simulink model "PQ_Control_LCL_4Legs"  (R2023b)
settings: Solver=FixedStepAuto  StartTime=0.0  StopTime=10.0  RelTol=1e-3
InitFcn:
  | Initialization_for_PQ_Control_LCL_4Legs;
values from neighbouring files (symbols this model uses):
  Fnom_Grid = 50    [Initialization_for_PQ_Control_LCL_4Legs.m]
  Gain_for_ActiveDamping = 1    [Initialization_for_PQ_Control_LCL_4Legs.m]
  Inom = Pnom/sqrt(3)/Unom_Grid    [Initialization_for_PQ_Control_LCL_4Legs.m]
  Ki_Idq = Kp_Idq*2*pi*0.5    (= 6.3165468167)    [Initialization_for_PQ_Control_LCL_4Legs.m]
  Ki_Un = Cdc/L_neutral*Kp_Un^2*Udc_ref/Inom    [Initialization_for_PQ_Control_LCL_4Legs.m]
  Kp_Idq = L_grid*2*pi*1600    (= 2.0106192983)    [Initialization_for_PQ_Control_LCL_4Legs.m]
  Kp_Un = 2*pi*Fnom_Grid*L_neutral*10    (= 1.13097335529)    [Initialization_for_PQ_Control_LCL_4Legs.m]
  L_grid = 200e-6    (= 0.0002)    [Initialization_for_PQ_Control_LCL_4Legs.m]
  Ts_Control = 62.5e-6    (= 6.25e-05)    [Initialization_for_PQ_Control_LCL_4Legs.m]
  Udc_ref = 1500    [Initialization_for_PQ_Control_LCL_4Legs.m]
  Unom_Phase = Unom_Grid/sqrt(3)    [Initialization_for_PQ_Control_LCL_4Legs.m]
libraries: LibraryForCodeGeneration x14
settings Model: DataDictionary=VariablesDictionary_for_PQ_Control_LCL_4Legs.sldd  TunableVars=Inom,Ki_Idq,Kp_Idq,Udc_ref,Unom_Phase  TunableVarsStorageClass=Auto,Auto,Auto,Auto,Auto  TunableVarsTypeQualifier=,,,,  Creator=ZZY  LastModifiedBy=ZZY
settings OptimizationCC: BlockReduction=off  DefaultParameterBehavior=Inlined  UseDivisionForNetSlopeComputation=on  ReuseModelBlockBuffer=off  ExpressionFolding=off  PassReuseOutputArgsAs=Individual arguments  ZeroExternalMemoryAtStartup=off  ZeroInternalMemoryAtStartup=off  EfficientFloat2IntCast=on  LifeSpan=inf  OptimizationLevel=level1  LabelGuidedReuse=on  EfficientTunableParamExpr=on
settings DebuggingCC: SignalInfNanChecking=warning  SignalRangeChecking=warning  ReadBeforeWriteMsg=EnableAllAsError  WriteAfterWriteMsg=EnableAllAsError  WriteAfterReadMsg=EnableAllAsError  IntegerOverflowMsg=error  ParameterPrecisionLossMsg=none  FixptConstUnderflowMsg=warning  FixptConstOverflowMsg=warning  FixptConstPrecisionLossMsg=warning  UnnecessaryDatatypeConvMsg=warning  UniqueDataStoreMsg=error  AssertControl=DisableAll  NonBusSignalsTreatedAsBus=error  SFInvalidInputDataAccessInChartInitDiag=error  SFTransitionOutsideNaturalParentDiag=error  SFUnreachableExecutionPathDiag=error  SFUndirectedBroadcastEventsDiag=error  IntegerSaturationMsg=error
settings HardwareCC: ProdBitPerChar=16  ProdBitPerInt=16  ProdBitPerPointer=32  ProdBitPerSizeT=32  ProdBitPerPtrDiffT=32  ProdLargestAtomicInteger=Integer  ProdLargestAtomicFloat=None  ProdWordSize=16  ProdHWDeviceType=Texas Instruments->C2000  TargetBitPerChar=16  TargetBitPerInt=16  TargetLargestAtomicInteger=Integer  TargetIntDivRoundTo=Zero  TargetEndianess=LittleEndian  TargetWordSize=16  TargetHWDeviceType=Texas Instruments->C2000
settings SFSimCC: CompileTimeRecursionLimit=0  EnableRuntimeRecursion=off  MATLABDynamicMemAlloc=off
settings RTWCC: Description=Embedded Coder  SystemTargetFile=ert.tlc  TemplateMakefile=ert_default_tmf  GenerateReport=on  Toolchain=MinGW64 | gmake (64-bit Windows)  BuildConfiguration=Faster Runs  IncludeHyperlinkInReport=on  LaunchReport=on  DataTypeReplacement=CDataTypesFixedWidth  GenerateTraceInfo=on  GenerateTraceReport=on  GenerateTraceReportSl=on  GenerateTraceReportSf=on  GenerateTraceReportEml=on  GenerateWebview=on  GenerateCodeReplacementReport=on  CheckMdlBeforeBuild=Warning
settings CodeAppCC: ForceParamTrailComments=on  IgnoreCustomStorageClasses=off  OperatorAnnotations=on  SimulinkDataObjDesc=on  SFDataObjDesc=on  MATLABFcnDesc=on  DefineNamingRule=UpperCase  InsertBlockDesc=on  StateflowObjectComments=on  MATLABSourceComments=on  InlinedPrmAccess=Macros  ReqsInCode=on
settings ERTTargetCC: TargetLangStandard=C99 (ISO)  GenerateSampleERTMain=on  CombineSignalStateStructs=on  GroupInternalDataByFunction=on  ParenthesesLevel=Standards  CastingMode=Standards  GenerateSharedConstants=off  ERTCustomFileTemplate=example_file_process.tlc  RateTransitionBlockCode=Function  PreserveExpressionOrder=on  PreserveIfCondition=on  ConvertIfToSwitch=off  SuppressUnreachableDefaultCases=off  EnableSignedLeftShifts=off  EnableSignedRightShifts=off  MaxIdInt64=INT64_MAX  MinIdInt64=INT64_MIN  MaxIdUint64=UINT64_MAX  MaxIdInt32=INT32_MAX  MinIdInt32=INT32_MIN  MaxIdUint32=UINT32_MAX  MaxIdInt16=INT16_MAX  MinIdInt16=INT16_MIN  MaxIdUint16=UINT16_MAX  MaxIdInt8=INT8_MAX  MinIdInt8=INT8_MIN  MaxIdUint8=UINT8_MAX

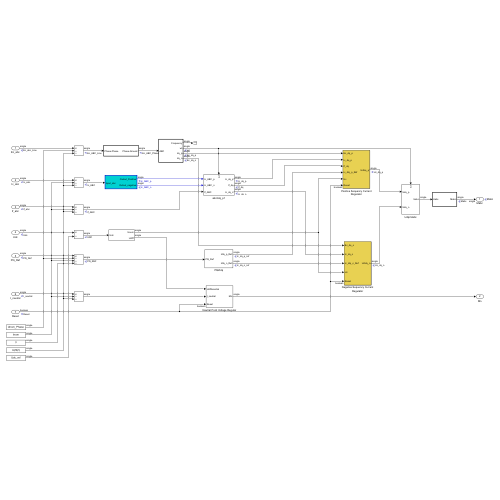
[thumbnail: Simulink's stored preview of the top-level diagram]
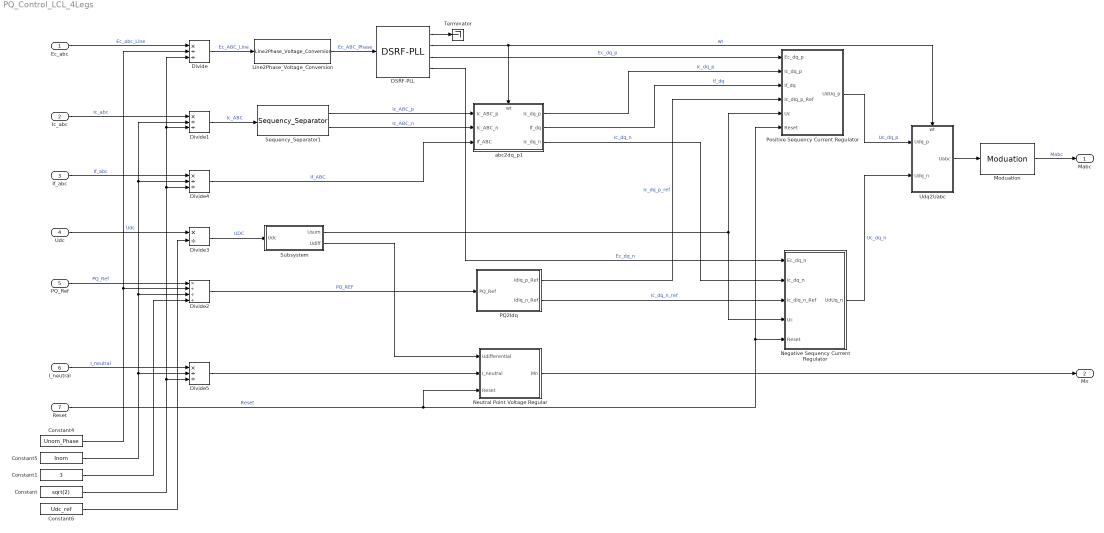
== system PQ_Control_LCL_4Legs ==
  Ec_abc : Inport  OutDataTypeStr=single
  Ic_abc : Inport  Port=2  OutDataTypeStr=single
  If_abc : Inport  Port=3  OutDataTypeStr=single
  Udc : Inport  Port=4  OutDataTypeStr=single
  PQ_Ref : Inport  Port=5  OutDataTypeStr=single
  I_neutral : Inport  Port=6  OutDataTypeStr=single
  Reset : Inport  Port=7  OutDataTypeStr=boolean
  Constant : Constant  Value=sqrt(2)  OutDataTypeStr=Inherit: Inherit via back propagation  SampleTime=-1
  Constant1 : Constant  Value=3  OutDataTypeStr=Inherit: Inherit via back propagation  SampleTime=-1
  Constant4 : Constant  Value=Unom_Phase  OutDataTypeStr=Inherit: Inherit via back propagation  SampleTime=-1
  Constant5 : Constant  Value=Inom  OutDataTypeStr=Inherit: Inherit via back propagation  SampleTime=-1
  Constant6 : Constant  Value=Udc_ref  OutDataTypeStr=Inherit: Inherit via back propagation  SampleTime=-1
  DSRF-PLL : LibraryForCodeGeneration/DSRF-PLL  Ts=Ts_Control
  Divide{,1,4..5} (4 alike) : Product  Inputs=*//  OutDataTypeStr=single
  Divide2 : Product  Inputs=*///  OutDataTypeStr=single
  Divide3 : Product  Inputs=*/  OutDataTypeStr=single
  Line2Phase_Voltage_Conversion : LibraryForCodeGeneration/Line2Phase_Voltage_Conversion  SystemSampleTime=-1  VariantActivationTime=update diagram  AllowFlexibleInterface=on  Latency=0  AutoFrameSizeCalculation=off
  Moduation : LibraryForCodeGeneration/Moduation  Modulation=SVPWM
  Negative Sequency Current Regulator : Subsystem
  Neutral Point Voltage Regular : Subsystem
  PQ2Idq : Subsystem
  Positive Sequency Current Regulator : Subsystem
  Sequency_Separator1 : LibraryForCodeGeneration/Sequency_Separator  SystemSampleTime=-1  VariantActivationTime=update diagram  AllowFlexibleInterface=on  Latency=0  AutoFrameSizeCalculation=off
  Subsystem : Subsystem
  Terminator : Terminator
  Udq2Uabc : Subsystem
      settings: PortSchema="{\"entries\":[{\"content\":{\"sides\":[{\"content\":{\"connectorIds\":[\"In1\",\"In2\"]},\"type\":\"ConnectorPlacement.EquallySpacedRectSide\",\"uuid\":\"009786f4-728c-4160-b9bf-eaf0b5a05101\"},{\"content\":{\"connectorIds\":[\"Out1\"],\"side\":\"RIGHT\"},\"type\":\"ConnectorPlacement.EquallySpacedRectSide\",\"uuid\":\"2a94367a-5c57-4632-9573-ab089470159a\"},{\"content\":{\"connectorIds\":[\"In3\"],\"side\":\"TOP\"},\"type\":\"ConnectorPlacement.EquallySpacedRectSide\",\"uuid\":\"6906365b-3187-4c4b-97cf-c9dec4c5ef7c\"}]},\"type\":\"ConnectorPlacement.EquallySpacedConnector\",\"uuid\":\"96ca8566-a266-405c-817a-b47b433d51ed\"}],\"packageUris\":[\"http://schema.mathworks.com/mf0/Connector/R2020b\"],\"version\":\"1.0\"}"
  abc2dq_p1 : Subsystem
      settings: PortSchema="{\"entries\":[{\"content\":{\"sides\":[{\"content\":{\"connectorIds\":[\"In1\",\"In2\",\"In3\"]},\"type\":\"ConnectorPlacement.EquallySpacedRectSide\",\"uuid\":\"702c7fae-dbbb-427d-af19-afd468018ae6\"},{\"content\":{\"connectorIds\":[\"Out1\",\"Out2\",\"Out3\"],\"side\":\"RIGHT\"},\"type\":\"ConnectorPlacement.EquallySpacedRectSide\",\"uuid\":\"d2ca5462-a446-46d8-bb73-1a455ffa959f\"},{\"content\":{\"connectorIds\":[\"In4\"],\"side\":\"TOP\"},\"type\":\"ConnectorPlacement.EquallySpacedRectSide\",\"uuid\":\"50bc6c44-424f-4342-960e-11540364fe97\"}]},\"type\":\"ConnectorPlacement.EquallySpacedConnector\",\"uuid\":\"f58cf64d-fe35-43f1-a031-7ee625a8bb1e\"}],\"packageUris\":[\"http://schema.mathworks.com/mf0/Connector/R2020b\"],\"version\":\"1.0\"}"
  Mabc : Outport  SignalName=Mabc  OutDataTypeStr=single
      settings: MustResolveToSignalObject=on
  Mn : Outport  Port=2
  wires:
  Line2Phase_Voltage_Conversion/1 -> DSRF-PLL/1  "Ec_ABC_Phase"
  Divide2/1 -> PQ2Idq/1(PQ_Ref)  "PQ_REF"
  PQ_Ref/1 -> Divide2/1  "PQ_Ref"
  Negative Sequency Current Regulator/1(UdUq_n) -> Udq2Uabc/2(Udq_n)  "Uc_dq_n"
  PQ2Idq/1(IdIq_p_Ref) -> Positive Sequency Current Regulator/4(Ic_dIq_p_Ref)  "Ic_dq_p_ref"
  abc2dq_p1/3(Ic_dq_n) -> Negative Sequency Current Regulator/2(Ic_dq_n)  "Ic_dq_n"
  Positive Sequency Current Regulator/1(UdUq_p) -> Udq2Uabc/1(Udq_p)  "Uc_dq_p"
  Divide3/1 -> Subsystem/1(Udc)  "UDC"
  DSRF-PLL/3 -> Positive Sequency Current Regulator/1(Ec_dq_p)  "Ec_dq_p"
  Ec_abc/1 -> Divide/1  "Ec_abc_Line"
  abc2dq_p1/1(Ic_dq_p) -> Positive Sequency Current Regulator/2(Ic_dq_p)  "Ic_dq_p"
  Divide1/1 -> Sequency_Separator1/1  "Ic_ABC"
  Ic_abc/1 -> Divide1/1  "Ic_abc"
  DSRF-PLL/4 -> Negative Sequency Current Regulator/1(Ec_dq_n)  "Ec_dq_n"
  Divide/1 -> Line2Phase_Voltage_Conversion/1  "Ec_ABC_Line"
  Udc/1 -> Divide3/1  "Udc"
  Udq2Uabc/1(Uabc) -> Moduation/1
  PQ2Idq/2(IdIq_n_Ref) -> Negative Sequency Current Regulator/3(Ic_dIq_n_Ref)  "Ic_dq_n_ref"
  Constant4/1 -> Divide/2, Divide2/2
  Constant/1 -> Divide4/3, Divide1/3, Divide/3, Divide5/3
  Constant5/1 -> Divide4/2, Divide1/2, Divide2/3, Divide5/2
  Constant1/1 -> Divide2/4
  Constant6/1 -> Divide3/2
  Reset/1 -> Positive Sequency Current Regulator/6(Reset), Negative Sequency Current Regulator/5(Reset), Neutral Point Voltage Regular/3(Reset)  "Reset"
  If_abc/1 -> Divide4/1  "If_abc"
  Divide4/1 -> abc2dq_p1/3(If_ABC)  "If_ABC"
  DSRF-PLL/2 -> Udq2Uabc/3(wt), abc2dq_p1/4(wt)  "wt"
  DSRF-PLL/1 -> Terminator/1
  Sequency_Separator1/2 -> abc2dq_p1/2("Ic_ABC_n ")  "Ic_ABC_n"
  Sequency_Separator1/1 -> abc2dq_p1/1("Ic_ABC_p ")  "Ic_ABC_p"
  abc2dq_p1/2(If_dq) -> Positive Sequency Current Regulator/3(If_dq)  "If_dq"
  Moduation/1 -> Mabc/1  "Mabc"
  Subsystem/1(Usum) -> Negative Sequency Current Regulator/4(Uc), Positive Sequency Current Regulator/5(Uc)
  Divide5/1 -> Neutral Point Voltage Regular/2(I_neutral)
  I_neutral/1 -> Divide5/1  "I_neutral"
  Subsystem/2(Udiff) -> Neutral Point Voltage Regular/1(Udifferential)
  Neutral Point Voltage Regular/1(Mn) -> Mn/1

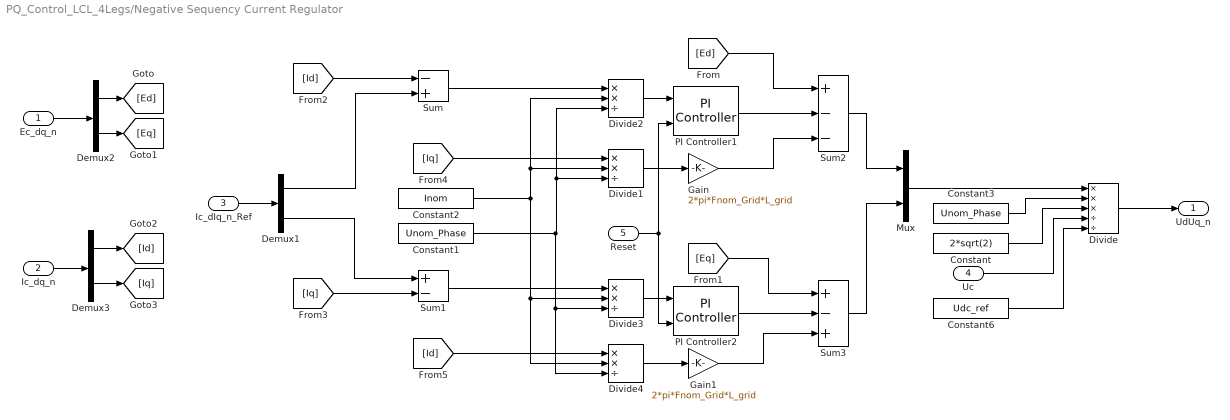
== system PQ_Control_LCL_4Legs/Negative Sequency Current Regulator ==
  Ec_dq_n : Inport
  Ic_dq_n : Inport  Port=2
  Ic_dIq_n_Ref : Inport  Port=3
  Uc : Inport  Port=4
  Reset : Inport  Port=5  OutDataTypeStr=boolean
  Constant : Constant  Value=2*sqrt(2)  OutDataTypeStr=Inherit: Inherit via back propagation  SampleTime=-1
  Constant1 : Constant  Value=Unom_Phase  OutDataTypeStr=Inherit: Inherit via back propagation  SampleTime=-1
  Constant2 : Constant  Value=Inom  OutDataTypeStr=Inherit: Inherit via back propagation  SampleTime=-1
  Constant3 : Constant  Value=Unom_Phase  OutDataTypeStr=Inherit: Inherit via back propagation  SampleTime=-1
  Constant6 : Constant  Value=Udc_ref  OutDataTypeStr=Inherit: Inherit via back propagation  SampleTime=-1
  Demux1 : Demux  Outputs=2
  Demux2 : Demux  Outputs=2
  Demux3 : Demux  Outputs=2
  Divide : Product  Inputs=***//  OutDataTypeStr=single
  Divide{1..4} (4 alike) : Product  Inputs=**/  OutDataTypeStr=single
  Gain : Gain  Gain=2*pi*Fnom_Grid*L_grid  ParamDataTypeStr=Inherit: Same as input
  Gain1 : Gain  Gain=2*pi*Fnom_Grid*L_grid  ParamDataTypeStr=Inherit: Same as input
  Mux : Mux  Inputs=2
  PI Controller1 : LibraryForCodeGeneration/PI Controller  Kp=Kp_Idq  Ki=Ki_Idq  Ts=Ts_Control  Max=2  Min=-2
  PI Controller2 : LibraryForCodeGeneration/PI Controller  Kp=Kp_Idq  Ki=Ki_Idq  Ts=Ts_Control  Max=2  Min=-2
  Sum : Sum  Inputs=-+  InputSameDT=on  SaturateOnIntegerOverflow=on  OutDataTypeStr=Inherit: Same as first input
  Sum1 : Sum  Inputs=+-  InputSameDT=on  SaturateOnIntegerOverflow=on  OutDataTypeStr=Inherit: Same as first input
  Sum2 : Sum  Inputs=+--  InputSameDT=on  SaturateOnIntegerOverflow=on  OutDataTypeStr=Inherit: Same as first input
  Sum3 : Sum  Inputs=+-+  InputSameDT=on  SaturateOnIntegerOverflow=on  OutDataTypeStr=Inherit: Same as first input
  UdUq_n : Outport
  wires:
  [Id] -> Divide4/1
  [Iq] -> Divide1/1
  [Iq] -> Sum1/2
  [Id] -> Sum/1
  Ic_dq_n/1 -> Demux3/1
  Demux3/1 -> [Id]
  Demux3/2 -> [Iq]
  Demux1/2 -> Sum1/1
  Demux1/1 -> Sum/2
  [Eq] -> Sum3/1
  [Ed] -> Sum2/1
  Demux2/2 -> [Eq]
  Demux2/1 -> [Ed]
  Divide3/1 -> PI Controller2/1
  Sum/1 -> Divide2/1
  Mux/1 -> Divide/1
  Divide/1 -> UdUq_n/1
  Gain1/1 -> Sum3/3
  Gain/1 -> Sum2/3
  Ec_dq_n/1 -> Demux2/1
  Ic_dIq_n_Ref/1 -> Demux1/1
  Sum2/1 -> Mux/1
  Sum1/1 -> Divide3/1
  Divide2/1 -> PI Controller1/1
  Sum3/1 -> Mux/2
  Reset/1 -> PI Controller2/2, PI Controller1/2
  Constant3/1 -> Divide/2
  Constant/1 -> Divide/3
  Uc/1 -> Divide/4
  Constant6/1 -> Divide/5
  Divide1/1 -> Gain/1
  Divide4/1 -> Gain1/1
  Constant2/1 -> Divide1/2, Divide2/2, Divide4/2, Divide3/2
  Constant1/1 -> Divide3/3, Divide4/3, Divide1/3, Divide2/3
  PI Controller2/1 -> Sum3/2
  PI Controller1/1 -> Sum2/2

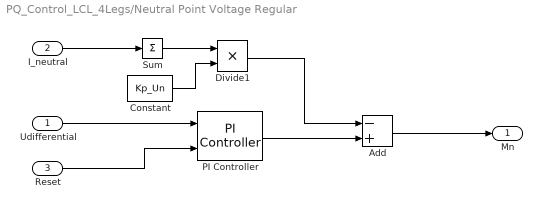
== system PQ_Control_LCL_4Legs/Neutral Point Voltage Regular ==
  Udifferential : Inport
  I_neutral : Inport  Port=2
  Reset : Inport  Port=3  OutDataTypeStr=boolean
  Add : Sum  Inputs=-+
  Constant : Constant  Value=Kp_Un  OutDataTypeStr=Inherit: Inherit via back propagation  SampleTime=-1
  Divide1 : Product  Inputs=**
  PI Controller : LibraryForCodeGeneration/PI Controller  Kp=1e-6  Ki=Ki_Un  Ts=Ts_Control  Max=1  Min=-1
  Sum : Sum  Inputs=+
  Mn : Outport
  wires:
  Add/1 -> Mn/1
  Reset/1 -> PI Controller/2
  Divide1/1 -> Add/1
  I_neutral/1 -> Sum/1
  PI Controller/1 -> Add/2
  Udifferential/1 -> PI Controller/1
  Constant/1 -> Divide1/2
  Sum/1 -> Divide1/1

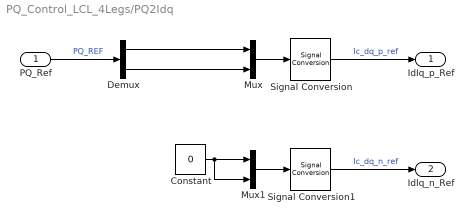
== system PQ_Control_LCL_4Legs/PQ2Idq ==
  PQ_Ref : Inport
  Constant : Constant  Value=0  OutDataTypeStr=Inherit: Inherit via back propagation  SampleTime=-1
  Demux : Demux  Outputs=2
  Mux : Mux  Inputs=2
  Mux1 : Mux  Inputs=2
  Signal Conversion : SignalConversion  OverrideOpt=off
  Signal Conversion1 : SignalConversion  OverrideOpt=off
  IdIq_p_Ref : Outport
  IdIq_n_Ref : Outport  Port=2
  wires:
  Mux1/1 -> Signal Conversion1/1
  Mux/1 -> Signal Conversion/1
  PQ_Ref/1 -> Demux/1  "PQ_REF"
  Demux/2 -> Mux/2
  Demux/1 -> Mux/1
  Signal Conversion/1 -> IdIq_p_Ref/1  "Ic_dq_p_ref"
  Signal Conversion1/1 -> IdIq_n_Ref/1  "Ic_dq_n_ref"
  Constant/1 -> Mux1/2, Mux1/1

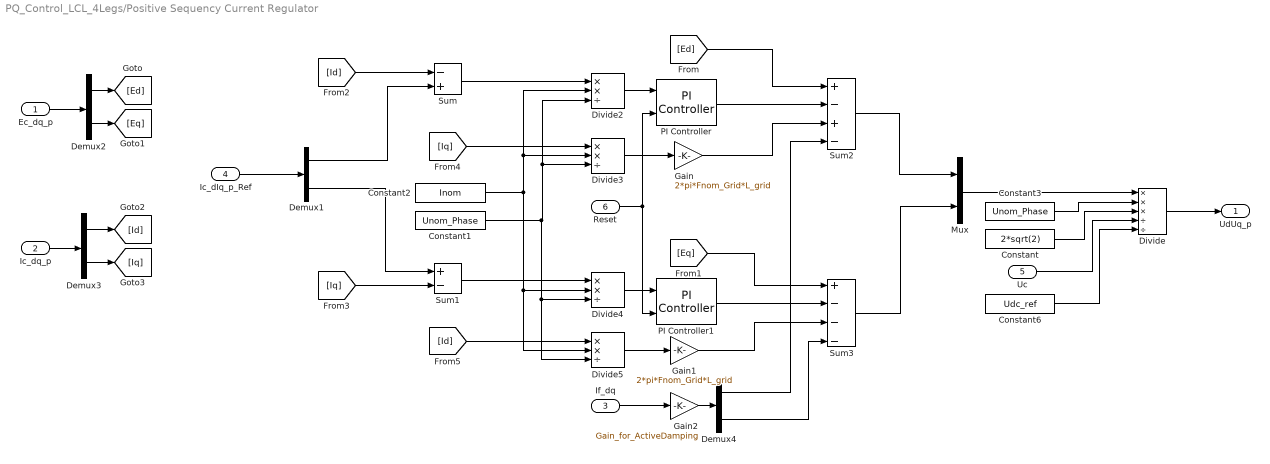
== system PQ_Control_LCL_4Legs/Positive Sequency Current Regulator ==
  Ec_dq_p : Inport
  Ic_dq_p : Inport  Port=2
  If_dq : Inport  Port=3
  Ic_dIq_p_Ref : Inport  Port=4
  Uc : Inport  Port=5
  Reset : Inport  Port=6  OutDataTypeStr=boolean
  Constant : Constant  Value=2*sqrt(2)  OutDataTypeStr=Inherit: Inherit via back propagation  SampleTime=-1
  Constant1 : Constant  Value=Unom_Phase  OutDataTypeStr=Inherit: Inherit via back propagation  SampleTime=-1
  Constant2 : Constant  Value=Inom  OutDataTypeStr=Inherit: Inherit via back propagation  SampleTime=-1
  Constant3 : Constant  Value=Unom_Phase  OutDataTypeStr=Inherit: Inherit via back propagation  SampleTime=-1
  Constant6 : Constant  Value=Udc_ref  OutDataTypeStr=Inherit: Inherit via back propagation  SampleTime=-1
  Demux{1..4} (4 alike) : Demux  Outputs=2
  Divide : Product  Inputs=***//  OutDataTypeStr=single
  Divide{2..5} (4 alike) : Product  Inputs=**/  OutDataTypeStr=single
  Gain : Gain  Gain=2*pi*Fnom_Grid*L_grid  ParamDataTypeStr=Inherit: Same as input
  Gain1 : Gain  Gain=2*pi*Fnom_Grid*L_grid  ParamDataTypeStr=Inherit: Same as input
  Gain2 : Gain  Gain=Gain_for_ActiveDamping  ParamDataTypeStr=Inherit: Same as input
  Mux : Mux  Inputs=2
  PI Controller : LibraryForCodeGeneration/PI Controller  Kp=Kp_Idq  Ki=Ki_Idq  Ts=Ts_Control  Max=2  Min=-2
  PI Controller1 : LibraryForCodeGeneration/PI Controller  Kp=Kp_Idq  Ki=Ki_Idq  Ts=Ts_Control  Max=2  Min=-2
  Sum : Sum  Inputs=-+  InputSameDT=on  SaturateOnIntegerOverflow=on  OutDataTypeStr=Inherit: Same as first input
  Sum1 : Sum  Inputs=+-  InputSameDT=on  SaturateOnIntegerOverflow=on  OutDataTypeStr=Inherit: Same as first input
  Sum2 : Sum  Inputs=+-+-  InputSameDT=on  SaturateOnIntegerOverflow=on  OutDataTypeStr=Inherit: Same as first input
  Sum3 : Sum  Inputs=+---  InputSameDT=on  SaturateOnIntegerOverflow=on  OutDataTypeStr=Inherit: Same as first input
  UdUq_p : Outport
  wires:
  Sum3/1 -> Mux/2
  Sum1/1 -> Divide4/1
  Sum2/1 -> Mux/1
  Ic_dIq_p_Ref/1 -> Demux1/1
  Uc/1 -> Divide/4
  Divide3/1 -> Gain/1
  Divide5/1 -> Gain1/1
  Ec_dq_p/1 -> Demux2/1
  Gain/1 -> Sum2/3
  Divide/1 -> UdUq_p/1
  Mux/1 -> Divide/1
  Sum/1 -> Divide2/1
  Divide4/1 -> PI Controller1/1
  Demux2/1 -> [Ed]
  Demux2/2 -> [Eq]
  [Ed] -> Sum2/1
  Demux1/1 -> Sum/2
  Demux1/2 -> Sum1/1
  Demux3/2 -> [Iq]
  Demux3/1 -> [Id]
  Ic_dq_p/1 -> Demux3/1
  [Id] -> Sum/1
  [Iq] -> Sum1/2
  [Iq] -> Divide3/1
  [Id] -> Divide5/1
  PI Controller/1 -> Sum2/2
  Divide2/1 -> PI Controller/1
  Reset/1 -> PI Controller1/2, PI Controller/2
  Constant3/1 -> Divide/2
  Constant/1 -> Divide/3
  Constant6/1 -> Divide/5
  Constant2/1 -> Divide5/2, Divide4/2, Divide3/2, Divide2/2
  Constant1/1 -> Divide5/3, Divide4/3, Divide3/3, Divide2/3
  If_dq/1 -> Gain2/1
  Demux4/1 -> Sum2/4
  Gain2/1 -> Demux4/1
  Demux4/2 -> Sum3/4
  [Eq] -> Sum3/1
  PI Controller1/1 -> Sum3/2
  Gain1/1 -> Sum3/3

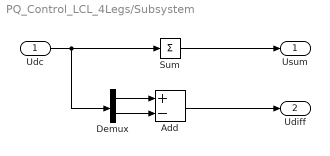
== system PQ_Control_LCL_4Legs/Subsystem ==
  Udc : Inport
  Add : Sum  Inputs=+-
  Demux : Demux  Outputs=2
  Sum : Sum  Inputs=+
  Usum : Outport
  Udiff : Outport  Port=2
  wires:
  Udc/1 -> Demux/1, Sum/1
  Sum/1 -> Usum/1
  Add/1 -> Udiff/1
  Demux/1 -> Add/1
  Demux/2 -> Add/2

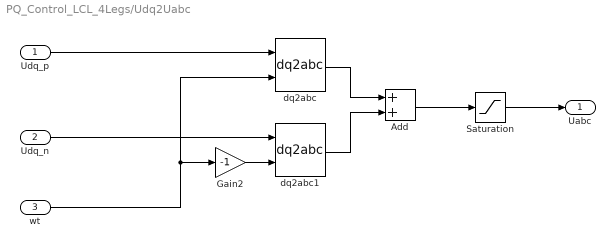
== system PQ_Control_LCL_4Legs/Udq2Uabc ==
  Udq_p : Inport
  Udq_n : Inport  Port=2
  wt : Inport  Port=3
  Add : Sum
  Gain2 : Gain  Gain=-1  ParamDataTypeStr=Inherit: Same as input
  Saturation : Saturate  UpperLimit=1.15  LowerLimit=-1.15
  dq2abc : LibraryForCodeGeneration/dq2abc  SystemSampleTime=-1  VariantActivationTime=update diagram  AllowFlexibleInterface=on  Latency=0  AutoFrameSizeCalculation=off
  dq2abc1 : LibraryForCodeGeneration/dq2abc  SystemSampleTime=-1  VariantActivationTime=update diagram  AllowFlexibleInterface=on  Latency=0  AutoFrameSizeCalculation=off
  Uabc : Outport
  wires:
  dq2abc1/1 -> Add/2
  wt/1 -> dq2abc/2, Gain2/1
  Gain2/1 -> dq2abc1/2
  Udq_p/1 -> dq2abc/1
  Udq_n/1 -> dq2abc1/1
  Add/1 -> Saturation/1
  dq2abc/1 -> Add/1
  Saturation/1 -> Uabc/1

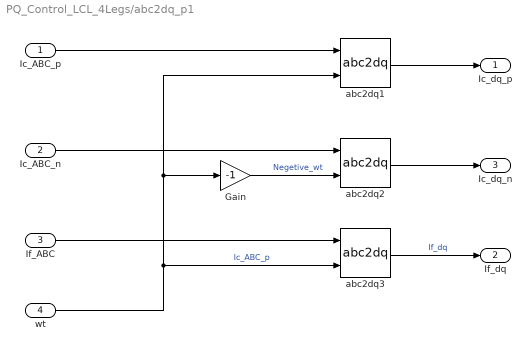
== system PQ_Control_LCL_4Legs/abc2dq_p1 ==
  "Ic_ABC_p " : Inport
  "Ic_ABC_n " : Inport  Port=2
  If_ABC : Inport  Port=3
  wt : Inport  Port=4
  Gain : Gain  Gain=-1
  abc2dq1 : LibraryForCodeGeneration/abc2dq  SystemSampleTime=-1  VariantActivationTime=update diagram  AllowFlexibleInterface=on  Latency=0  AutoFrameSizeCalculation=off
  abc2dq2 : LibraryForCodeGeneration/abc2dq  SystemSampleTime=-1  VariantActivationTime=update diagram  AllowFlexibleInterface=on  Latency=0  AutoFrameSizeCalculation=off
  abc2dq3 : LibraryForCodeGeneration/abc2dq  SystemSampleTime=-1  VariantActivationTime=update diagram  AllowFlexibleInterface=on  Latency=0  AutoFrameSizeCalculation=off
  Ic_dq_p : Outport
  If_dq : Outport  Port=2
  Ic_dq_n : Outport  Port=3
  wires:
  "Ic_ABC_p "/1 -> abc2dq1/1
  abc2dq1/1 -> Ic_dq_p/1
  If_ABC/1 -> abc2dq3/1
  abc2dq3/1 -> If_dq/1  "If_dq"
  Gain/1 -> abc2dq2/2  "Negetive_wt"
  "Ic_ABC_n "/1 -> abc2dq2/1
  abc2dq2/1 -> Ic_dq_n/1
  wt/1 -> abc2dq1/2, Gain/1, abc2dq3/2  "Ic_ABC_p"
